simulink model "Quadcopter_State_model_Arduino"  (R2023b)
settings: Solver=VariableStepAuto  StartTime=0.0  StopTime=inf  FixedStep=0.00001  MinStep=0.001  RelTol=1e-3
model workspace (MAT data in the model file):
  DesiredPitchRoll : sugfis (value not decoded)
  DesiredThrust : sugfis (value not decoded)
  DesiredYaw : sugfis (value not decoded)
  Desired_Pitch = 0
  Desired_Roll = 0
  Desired_Yaw = 0
  Desired_Z_Velocity = -3
  FuzzyMotorspeed : sugfis (value not decoded)
values from neighbouring files (symbols this model uses):
  g = 9.81    [Quadcopter_Constants.m]
  Ixx = 0.0294838    [Quadcopter_Constants.m]
  Iyy = 0.0294838    [Quadcopter_Constants.m]
  Izz = 0.058967624    [Quadcopter_Constants.m]
  Jr = (6e-5)*1.358    (= 8.148e-05)    [Quadcopter_Constants.m]
  kd = 1    [Quadcopter_Constants.m]
  kd_phi = 1    [Quadcopter_Constants.m]
  kd_theta = 1    [Quadcopter_Constants.m]
  kf = 1    [Quadcopter_Constants.m]
  ki = 1    [Quadcopter_Constants.m]
  ki_phi = 1    [Quadcopter_Constants.m]
  ki_theta = 1    [Quadcopter_Constants.m]
  km = 4.74157e-9    (= 4.74157e-09)    [Quadcopter_Constants.m]
  kp = 1    [Quadcopter_Constants.m]
  kp_phi = 1    [Quadcopter_Constants.m]
  kp_theta = 1    [Quadcopter_Constants.m]
  kr = (0.1)*1.358    (= 0.1358)    [Quadcopter_Constants.m]
  kt = (0.1)*1.358    (= 0.1358)    [Quadcopter_Constants.m]
  l = 0.254    [Quadcopter_Constants.m]
  m = 0.914    [Quadcopter_Constants.m]
  sample_freq = 1000    [Quadcopter_Constants.m]
undefined symbols (not defined in the file or in its folder): LF
libraries: fuzblock x18, instrumentseriallib x12, simulink_extras x6, vrlib x4, instrumentlib x3, etargetslib x1, slpidlib x1, simulink x1
(part 4 of 5)

== system Quadcopter_State_model_Arduino/Board Fuzzy Only/Fuzzy Control System/Heading Controller ==
  <psi> : Inport
  <psi_dot> : Inport  Port=2
  Bus Creator2 : BusCreator  Inputs=2
  Desired Yaw2 : Constant  Value=Desired_Yaw
  DesiredYaw : fuzblock/Fuzzy Logic  Controller  FIS=DesiredYaw  OutputSampleNumber=101  DataType=double  FuzzifiedInputs=off  RuleFiringStrengths=off  RuleOutputs=off  AggregatedOutputs=off  SimulateUsing=Interpreted execution  OutOfRangeInputValueMessage=warning  NoRuleFiredMessage=warning  EmptyOutputFuzzySetMessage=warning
  Sum3 : Sum  Inputs=|-+
  e_yaw_sat : Saturate  UpperLimit=0.3  LowerLimit=-0.3  OutMin=[-0.3]  OutMax=[0.3]
  psidot_sat : Saturate  UpperLimit=0.3  LowerLimit=-0.3  OutMin=[-0.3]  OutMax=[0.3]
  Desired Yaw1 : Outport
  wires:
  psidot_sat/1 -> Bus Creator2/2
  <psi_dot>/1 -> psidot_sat/1
  Desired Yaw2/1 -> Sum3/2
  e_yaw_sat/1 -> Bus Creator2/1
  <psi>/1 -> Sum3/1
  DesiredYaw/1 -> Desired Yaw1/1  "Desired Yaw"
  Sum3/1 -> e_yaw_sat/1  "e_yaw"
  Bus Creator2/1 -> DesiredYaw/1

== system Quadcopter_State_model_Arduino/Board Fuzzy Only/Fuzzy Control System/Thrust Controller ==
  <z_dot> : Inport
  Desired Thrust : fuzblock/Fuzzy Logic  Controller  FIS=DesiredThrust  OutputSampleNumber=101  DataType=double  FuzzifiedInputs=off  RuleFiringStrengths=off  RuleOutputs=off  AggregatedOutputs=off  SimulateUsing=Interpreted execution  OutOfRangeInputValueMessage=warning  NoRuleFiredMessage=warning  EmptyOutputFuzzySetMessage=warning
  Desired Z Velocity1 : Constant  Value=Desired_Z_Velocity
  Sum : Sum  Inputs=|-+
  e_zdot_sat : Saturate  UpperLimit=0.3  LowerLimit=-0.3  OutMin=[-0.3]  OutMax=[0.3]
  Desired Thrust1 : Outport
  wires:
  Sum/1 -> e_zdot_sat/1  "e_zdot"
  <z_dot>/1 -> Sum/1
  Desired Z Velocity1/1 -> Sum/2
  e_zdot_sat/1 -> Desired Thrust/1
  Desired Thrust/1 -> Desired Thrust1/1  "Desired Thrust"

== system Quadcopter_State_model_Arduino/Board Fuzzy Only/Fuzzy Control System1/Attitude Controller ==
  <phi> : Inport
  <phi_dot> : Inport  Port=2
  <theta> : Inport  Port=3
  <theta_dot> : Inport  Port=4
  Bus Creator1 : BusCreator  Inputs=4
  Demux1 : Demux  Outputs=2
  Desired Pitch2 : Constant  Value=Desired_Pitch
  Desired Roll2 : Constant  Value=Desired_Roll
  DesiredPitchRoll : fuzblock/Fuzzy Logic  Controller  FIS=DesiredPitchRoll  OutputSampleNumber=101  DataType=double  FuzzifiedInputs=off  RuleFiringStrengths=off  RuleOutputs=off  AggregatedOutputs=off  SimulateUsing=Interpreted execution  OutOfRangeInputValueMessage=warning  NoRuleFiredMessage=warning  EmptyOutputFuzzySetMessage=warning
  Sum1 : Sum  Inputs=|-+
  Sum2 : Sum  Inputs=|-+
  e_pitch_sat : Saturate  UpperLimit=0.3  LowerLimit=-0.3  OutMin=[-0.3]  OutMax=[0.3]
  e_roll_sat : Saturate  UpperLimit=0.3  LowerLimit=-0.3  OutMin=[-0.3]  OutMax=[0.3]
  phidot_sat1 : Saturate  UpperLimit=0.3  LowerLimit=-0.3  OutMin=[-0.3]  OutMax=[0.3]
  thetadot_sat : Saturate  UpperLimit=0.3  LowerLimit=-0.3  OutMin=[-0.3]  OutMax=[0.3]
  Desired Roll1 : Outport
  Desired Pitch1 : Outport  Port=2
  wires:
  e_roll_sat/1 -> Bus Creator1/1
  phidot_sat1/1 -> Bus Creator1/4
  Sum2/1 -> e_pitch_sat/1  "e_pitch"
  Desired Roll2/1 -> Sum1/2
  e_pitch_sat/1 -> Bus Creator1/2
  DesiredPitchRoll/1 -> Demux1/1
  Bus Creator1/1 -> DesiredPitchRoll/1
  Demux1/2 -> Desired Pitch1/1  "Desired Pitch"
  Desired Pitch2/1 -> Sum2/2
  Sum1/1 -> e_roll_sat/1  "e_roll"
  thetadot_sat/1 -> Bus Creator1/3
  <phi>/1 -> Sum2/1
  <theta>/1 -> Sum1/1
  Demux1/1 -> Desired Roll1/1  "Desired Roll"
  <phi_dot>/1 -> phidot_sat1/1
  <theta_dot>/1 -> thetadot_sat/1

== system Quadcopter_State_model_Arduino/Board Fuzzy Only/Fuzzy Control System1/Heading Controller ==
  <psi> : Inport
  <psi_dot> : Inport  Port=2
  Bus Creator2 : BusCreator  Inputs=2
  Desired Yaw2 : Constant  Value=Desired_Yaw
  DesiredYaw : fuzblock/Fuzzy Logic  Controller  FIS=DesiredYaw  OutputSampleNumber=101  DataType=double  FuzzifiedInputs=off  RuleFiringStrengths=off  RuleOutputs=off  AggregatedOutputs=off  SimulateUsing=Interpreted execution  OutOfRangeInputValueMessage=warning  NoRuleFiredMessage=warning  EmptyOutputFuzzySetMessage=warning
  Sum3 : Sum  Inputs=|-+
  e_yaw_sat : Saturate  UpperLimit=0.3  LowerLimit=-0.3  OutMin=[-0.3]  OutMax=[0.3]
  psidot_sat : Saturate  UpperLimit=0.3  LowerLimit=-0.3  OutMin=[-0.3]  OutMax=[0.3]
  Desired Yaw1 : Outport
  wires:
  psidot_sat/1 -> Bus Creator2/2
  <psi_dot>/1 -> psidot_sat/1
  Desired Yaw2/1 -> Sum3/2
  e_yaw_sat/1 -> Bus Creator2/1
  <psi>/1 -> Sum3/1
  DesiredYaw/1 -> Desired Yaw1/1  "Desired Yaw"
  Sum3/1 -> e_yaw_sat/1  "e_yaw"
  Bus Creator2/1 -> DesiredYaw/1

== system Quadcopter_State_model_Arduino/Board Fuzzy Only/Fuzzy Control System1/MMA ==
  Desired Thrust1 : Inport
  Desired Yaw1 : Inport  Port=2
  Desired Pitch1 : Inport  Port=3
  Desired Roll1 : Inport  Port=4
  Bus Creator : BusCreator  Inputs=4
  motorspeeds : Outport
  wires:
  Bus Creator/1 -> motorspeeds/1

== system Quadcopter_State_model_Arduino/Board Fuzzy Only/Fuzzy Control System1/Thrust Controller ==
  <z_dot> : Inport
  Desired Thrust : fuzblock/Fuzzy Logic  Controller  FIS=DesiredThrust  OutputSampleNumber=101  DataType=double  FuzzifiedInputs=off  RuleFiringStrengths=off  RuleOutputs=off  AggregatedOutputs=off  SimulateUsing=Interpreted execution  OutOfRangeInputValueMessage=warning  NoRuleFiredMessage=warning  EmptyOutputFuzzySetMessage=warning
  Desired Z Velocity1 : Constant  Value=Desired_Z_Velocity
  Sum : Sum  Inputs=|-+
  e_zdot_sat : Saturate  UpperLimit=2.99999  LowerLimit=-2.99999
  Desired Thrust1 : Outport
  wires:
  Sum/1 -> e_zdot_sat/1  "e_zdot"
  <z_dot>/1 -> Sum/1
  Desired Z Velocity1/1 -> Sum/2
  e_zdot_sat/1 -> Desired Thrust/1
  Desired Thrust/1 -> Desired Thrust1/1  "Desired Thrust"

== system Quadcopter_State_model_Arduino/Board Fuzzy Only/Fuzzy Control System2/Attitude Error ==
  <phi> : Inport
  <phi_dot> : Inport  Port=2
  <theta> : Inport  Port=3
  <theta_dot> : Inport  Port=4
  Desired Pitch2 : Constant  Value=0
  Desired Roll2 : Constant  Value=0
  Sum1 : Sum  Inputs=|-+
  Sum2 : Sum  Inputs=|-+
  e_pitch_sat : Saturate  UpperLimit=0.3  LowerLimit=-0.3  OutMin=[-0.3]  OutMax=[0.3]
  e_roll_sat : Saturate  UpperLimit=0.3  LowerLimit=-0.3  OutMin=[-0.3]  OutMax=[0.3]
  phidot_sat1 : Saturate  UpperLimit=0.3  LowerLimit=-0.3  OutMin=[-0.3]  OutMax=[0.3]
  thetadot_sat : Saturate  UpperLimit=0.3  LowerLimit=-0.3  OutMin=[-0.3]  OutMax=[0.3]
  Out1 : Outport
  Out2 : Outport  Port=2
  Out3 : Outport  Port=3
  Out4 : Outport  Port=4
  wires:
  <phi>/1 -> Sum2/1
  Sum2/1 -> e_pitch_sat/1  "e_pitch"
  Desired Pitch2/1 -> Sum2/2
  <phi_dot>/1 -> phidot_sat1/1
  Desired Roll2/1 -> Sum1/2
  Sum1/1 -> e_roll_sat/1  "e_roll"
  e_pitch_sat/1 -> Out2/1
  <theta_dot>/1 -> thetadot_sat/1
  e_roll_sat/1 -> Out1/1
  <theta>/1 -> Sum1/1
  thetadot_sat/1 -> Out3/1
  phidot_sat1/1 -> Out4/1

== system Quadcopter_State_model_Arduino/Board Fuzzy Only/Fuzzy Control System2/Heading Error ==
  In1 : Inport
  In2 : Inport  Port=2
  Desired Yaw2 : Constant  Value=0
  Sum3 : Sum  Inputs=|-+
  e_yaw_sat : Saturate  UpperLimit=0.3  LowerLimit=-0.3  OutMin=[-0.3]  OutMax=[0.3]
  psidot_sat : Saturate  UpperLimit=0.3  LowerLimit=-0.3  OutMin=[-0.3]  OutMax=[0.3]
  Out1 : Outport
  Out2 : Outport  Port=2
  wires:
  Desired Yaw2/1 -> Sum3/2
  Sum3/1 -> e_yaw_sat/1  "e_yaw"
  In1/1 -> Sum3/1
  e_yaw_sat/1 -> Out1/1
  psidot_sat/1 -> Out2/1
  In2/1 -> psidot_sat/1

== system Quadcopter_State_model_Arduino/Board Fuzzy Only/Fuzzy Control System2/Subsystem ==
  In1 : Inport
  In2 : Inport  Port=2
  Bus Creator1 : BusCreator  Inputs=4
  Demux1 : Demux
  Divide{,1..3} (4 alike) : Product  Inputs=*/
  Gain4 : Gain  Gain=4
  Product{,1..3} (4 alike) : Product
  Scope : Scope  NumInputPorts=4
  Scope1 : Scope  NumInputPorts=4
  Sum : Sum  Inputs=++++  OutDataTypeStr=double  AccumDataTypeStr=double
  Out1 : Outport
  wires:
  In2/1 -> Gain4/1
  Demux1/2 -> Sum/2, Scope/2, Divide3/1  "Omega2"
  Divide1/1 -> Product3/1
  Sum/1 -> Divide1/2, Divide2/2, Divide3/2, Divide/2
  Demux1/1 -> Sum/1, Divide/1, Scope/1  "Omega1"
  Demux1/4 -> Sum/4, Scope/4, Divide1/1  "Omega4"
  Divide3/1 -> Product1/1
  Divide/1 -> Product/1
  Bus Creator1/1 -> Out1/1
  Demux1/3 -> Scope/3, Divide2/1, Sum/3  "Omega3"
  Divide2/1 -> Product2/1
  In1/1 -> Demux1/1
  Product/1 -> Scope1/1, Bus Creator1/1
  Product1/1 -> Scope1/2, Bus Creator1/2
  Product2/1 -> Scope1/3, Bus Creator1/3
  Product3/1 -> Scope1/4, Bus Creator1/4
  Gain4/1 -> Product3/2, Product2/2, Product1/2, Product/2

== system Quadcopter_State_model_Arduino/Board Fuzzy Only/Fuzzy Control System2/Zdot Error ==
  In1 : Inport
  Desired Z Velocity1 : Constant  Value=0
  Sum : Sum  Inputs=|-+
  e_zdot_sat : Saturate  UpperLimit=3  LowerLimit=-3  OutMin=[-3]  OutMax=[3]
  Out1 : Outport
  wires:
  In1/1 -> Sum/1
  Sum/1 -> e_zdot_sat/1  "e_zdot"
  Desired Z Velocity1/1 -> Sum/2
  e_zdot_sat/1 -> Out1/1

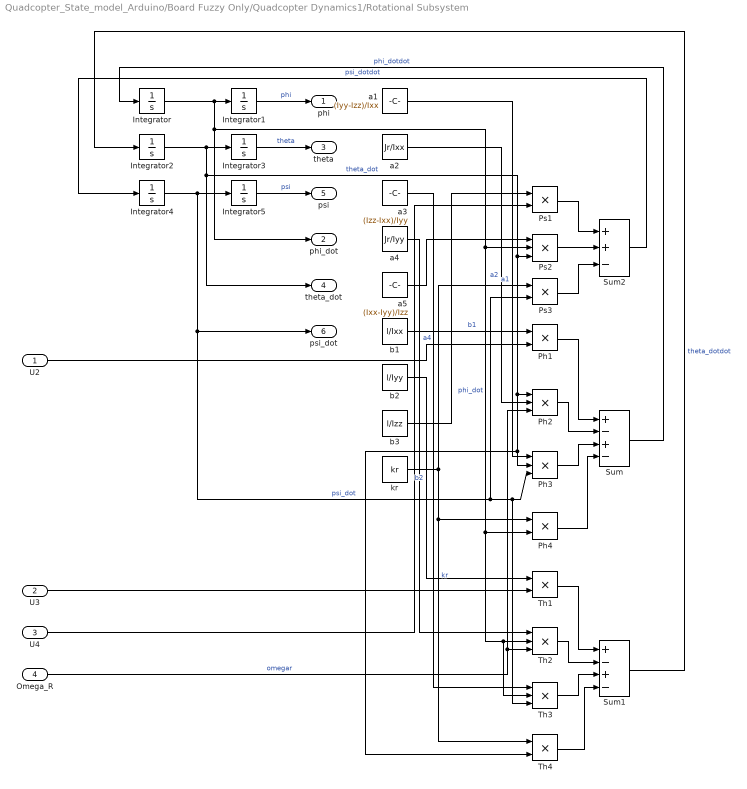
== system Quadcopter_State_model_Arduino/Board Fuzzy Only/Quadcopter Dynamics1/Rotational Subsystem ==
  U2 : Inport
  U3 : Inport  Port=2
  U4 : Inport  Port=3
  Omega_R : Inport  Port=4
  Integrator{,1..5} (6 alike) : Integrator
  Ph1 : Product
  Ph2 : Product  Inputs=3
  Ph3 : Product  Inputs=3
  Ph4 : Product
  Ps1 : Product
  Ps2 : Product  Inputs=3
  Ps3 : Product
  Sum : Sum  Inputs=+-+-
  Sum1 : Sum  Inputs=+-+-
  Sum2 : Sum  Inputs=++-
  Th1 : Product
  Th2 : Product  Inputs=3
  Th3 : Product  Inputs=3
  Th4 : Product
  a1 : Constant  Value=(Iyy-Izz)/Ixx
  a2 : Constant  Value=Jr/Ixx
  a3 : Constant  Value=(Izz-Ixx)/Iyy
  a4 : Constant  Value=Jr/Iyy
  a5 : Constant  Value=(Ixx-Iyy)/Izz
  b1 : Constant  Value=l/Ixx
  b2 : Constant  Value=l/Iyy
  b3 : Constant  Value=l/Izz
  kr : Constant  Value=kr
  phi : Outport
  phi_dot : Outport  Port=2
  theta : Outport  Port=3
  theta_dot : Outport  Port=4
  psi : Outport  Port=5
  psi_dot : Outport  Port=6
  wires:
  U4/1 -> Ps1/2
  Ph3/1 -> Sum/3
  kr/1 -> Ps3/1, Ph4/1, Th4/1  "kr"
  Th1/1 -> Sum1/1
  Sum/1 -> Integrator/1  "phi_dotdot"
  Omega_R/1 -> Ph2/3, Th2/3  "omegar"
  Th2/1 -> Sum1/2
  Integrator4/1 -> Integrator5/1, psi_dot/1, Ps3/2, Th3/3, Ph3/3  "psi_dot"
  Integrator2/1 -> Integrator3/1, theta_dot/1, Ps2/3, Ph3/2, Th4/2, Ph2/1  "theta_dot"
  Th3/1 -> Sum1/3
  a4/1 -> Th2/1  "a4"
  Sum2/1 -> Integrator4/1  "psi_dotdot"
  Integrator1/1 -> phi/1  "phi"
  U2/1 -> Ph1/2
  Sum1/1 -> Integrator2/1  "theta_dotdot"
  Integrator/1 -> phi_dot/1, Ps2/2, Ph4/2, Th3/2, Th2/2, Integrator1/1  "phi_dot"
  Th4/1 -> Sum1/4
  Integrator3/1 -> theta/1  "theta"
  b1/1 -> Ph1/1  "b1"
  a3/1 -> Th3/1
  b3/1 -> Ps1/1
  a2/1 -> Ph2/2  "a2"
  a1/1 -> Ph3/1  "a1"
  a5/1 -> Ps2/1
  U3/1 -> Th1/2
  Ps3/1 -> Sum2/3
  Ps1/1 -> Sum2/1
  Ps2/1 -> Sum2/2
  Ph4/1 -> Sum/4
  b2/1 -> Th1/1  "b2"
  Ph1/1 -> Sum/1
  Ph2/1 -> Sum/2
  Integrator5/1 -> psi/1  "psi"

== system Quadcopter_State_model_Arduino/Board Fuzzy Only/Quadcopter Dynamics1/Translational Subsystem 2.0 ==
  U1 : Inport
  phi : Inport  Port=2
  theta : Inport  Port=3
  psi : Inport  Port=4
  FWx : Inport  Port=5
  FWy : Inport  Port=6
  FWz : Inport  Port=7
  Integrator{6..11} (6 alike) : Integrator
  x_dotdot : Subsystem
      settings: PortSchema="{\"entries\":[{\"content\":{\"sides\":[{\"content\":{\"connectorIds\":[\"In1\",\"In2\",\"In3\",\"In4\",\"In5\",\"In6\",\"In7\"]},\"type\":\"ConnectorPlacement.EquallySpacedRectSide\",\"uuid\":\"e18be740-6f58-4938-bfd9-cb9ac7dcd4da\"},{\"content\":{\"connectorIds\":[\"In8\",\"Out1\"],\"side\":\"RIGHT\"},\"type\":\"ConnectorPlacement.EquallySpacedRectSide\",\"uuid\":\"68bb1cbd-6e96-465a-bd08-5b84ec49c8af\"},{\"content\":{\"connectorIds\":[],\"side\":\"TOP\"},\"type\":\"ConnectorPlacement.EquallySpacedRectSide\",\"uuid\":\"38ea75c0-d618-4b9d-8119-0da292fc369a\"}]},\"type\":\"ConnectorPlacement.EquallySpacedConnector\",\"uuid\":\"3f5248e6-8959-4c7a-b37c-028caf22ec16\"}],\"packageUris\":[\"http://schema.mathworks.com/mf0/Connector/R2020b\"],\"version\":\"1.0\"}"
  y_dotdot : Subsystem
      settings: PortSchema="{\"entries\":[{\"content\":{\"sides\":[{\"content\":{\"connectorIds\":[\"In1\",\"In2\",\"In3\",\"In4\",\"In5\",\"In6\",\"In7\"]},\"type\":\"ConnectorPlacement.EquallySpacedRectSide\",\"uuid\":\"e18be740-6f58-4938-bfd9-cb9ac7dcd4da\"},{\"content\":{\"connectorIds\":[\"In8\",\"Out1\"],\"side\":\"RIGHT\"},\"type\":\"ConnectorPlacement.EquallySpacedRectSide\",\"uuid\":\"68bb1cbd-6e96-465a-bd08-5b84ec49c8af\"},{\"content\":{\"connectorIds\":[],\"side\":\"TOP\"},\"type\":\"ConnectorPlacement.EquallySpacedRectSide\",\"uuid\":\"38ea75c0-d618-4b9d-8119-0da292fc369a\"}]},\"type\":\"ConnectorPlacement.EquallySpacedConnector\",\"uuid\":\"3f5248e6-8959-4c7a-b37c-028caf22ec16\"}],\"packageUris\":[\"http://schema.mathworks.com/mf0/Connector/R2020b\"],\"version\":\"1.0\"}"
  z_dodot : Subsystem
      settings: PortSchema="{\"entries\":[{\"content\":{\"sides\":[{\"content\":{\"connectorIds\":[\"In1\",\"In2\",\"In3\",\"In4\",\"In5\",\"In6\"]},\"type\":\"ConnectorPlacement.EquallySpacedRectSide\",\"uuid\":\"469c81c2-5293-4bed-8306-2e0ffdc3049a\"},{\"content\":{\"connectorIds\":[\"In7\",\"Out1\"],\"side\":\"RIGHT\"},\"type\":\"ConnectorPlacement.EquallySpacedRectSide\",\"uuid\":\"eb4ccd77-d780-4218-b458-09af15aced4a\"},{\"content\":{\"connectorIds\":[],\"side\":\"TOP\"},\"type\":\"ConnectorPlacement.EquallySpacedRectSide\",\"uuid\":\"6490e6c2-4333-4700-a2fe-e5c918a55a4d\"}]},\"type\":\"ConnectorPlacement.EquallySpacedConnector\",\"uuid\":\"88d53b3a-6da6-4ffe-908b-5dd465569eed\"}],\"packageUris\":[\"http://schema.mathworks.com/mf0/Connector/R2020b\"],\"version\":\"1.0\"}"
  x : Outport
  x_dot : Outport  Port=2
  y : Outport  Port=3
  y_dot : Outport  Port=4
  z : Outport  Port=5
  z_dot : Outport  Port=6
  wires:
  Integrator10/1 -> z_dot/1, z_dodot/7(z_dot), Integrator11/1  "z_dot"
  Integrator8/1 -> Integrator9/1, y_dotdot/8(y_dot), y_dot/1  "y_dot"
  Integrator9/1 -> y/1  "y"
  Integrator7/1 -> x/1  "x"
  Integrator6/1 -> x_dotdot/8(x_dot), x_dot/1, Integrator7/1  "x_dot"
  Integrator11/1 -> z/1  "z"
  U1/1 -> z_dodot/1(U1), y_dotdot/1(U1), x_dotdot/1(U1)  "U1"
  phi/1 -> y_dotdot/2(phi), x_dotdot/2(phi), z_dodot/2(phi)  "Phi"
  theta/1 -> z_dodot/3(theta), y_dotdot/3(theta), x_dotdot/3(theta)  "Theta"
  psi/1 -> y_dotdot/4(psi), x_dotdot/4(psi)  "Psi"
  FWx/1 -> z_dodot/4(FWx), y_dotdot/5(FWx), x_dotdot/5(FWx)  "FWx"
  FWy/1 -> z_dodot/5(FWy), y_dotdot/6(FWy), x_dotdot/6(FWy)  "FWy"
  FWz/1 -> z_dodot/6(FWz), y_dotdot/7(FWz), x_dotdot/7(FWz)  "FWz"
  z_dodot/1(z_dotdot) -> Integrator10/1
  y_dotdot/1(y_dotdot) -> Integrator8/1
  x_dotdot/1(x_dotdot) -> Integrator6/1

== system Quadcopter_State_model_Arduino/Board Fuzzy Only/Quadcopter Dynamics1/Translational Wind Engine ==
  phi : Inport
  theta : Inport  Port=2
  psi : Inport  Port=3
  Projected Areas : Subsystem
  Wind Forces : Subsystem
  Wind Generation : Subsystem
  FWx : Outport
  FWy : Outport  Port=2
  FWz : Outport  Port=3
  wires:
  theta/1 -> Projected Areas/1(theta)
  Wind Generation/3(VWz) -> Wind Forces/6(VWz)
  Projected Areas/3(Az) -> Wind Forces/3(Az)
  Wind Forces/3(FWz) -> FWz/1
  Wind Generation/2(VWy) -> Wind Forces/5(VWy)
  Projected Areas/1(Ax) -> Wind Forces/1(Ax)
  Projected Areas/2(Ay) -> Wind Forces/2(Ay)
  Wind Generation/1(VWx) -> Wind Forces/4(VWx)
  phi/1 -> Projected Areas/3(phi)
  psi/1 -> Projected Areas/2(psi)
  Wind Forces/2(FWy) -> FWy/1
  Wind Forces/1(FWx) -> FWx/1

== system Quadcopter_State_model_Arduino/Fuzzy Simulation/Fuzzy Control System/Attitude Controller ==
  <phi> : Inport
  <phi_dot> : Inport  Port=2
  <theta> : Inport  Port=3
  <theta_dot> : Inport  Port=4
  Bus Creator1 : BusCreator  Inputs=4
  Demux1 : Demux  Outputs=2
  Desired Pitch2 : Constant  Value=Desired_Pitch
  Desired Roll2 : Constant  Value=Desired_Roll
  DesiredPitchRoll : fuzblock/Fuzzy Logic  Controller  FIS=DesiredPitchRoll  OutputSampleNumber=101  DataType=double  FuzzifiedInputs=off  RuleFiringStrengths=off  RuleOutputs=off  AggregatedOutputs=off  SimulateUsing=Interpreted execution  OutOfRangeInputValueMessage=warning  NoRuleFiredMessage=warning  EmptyOutputFuzzySetMessage=warning
  Sum1 : Sum  Inputs=|-+
  Sum2 : Sum  Inputs=|-+
  e_pitch_sat : Saturate  UpperLimit=0.3  LowerLimit=-0.3  OutMin=[-0.3]  OutMax=[0.3]
  e_roll_sat : Saturate  UpperLimit=0.3  LowerLimit=-0.3  OutMin=[-0.3]  OutMax=[0.3]
  phidot_sat1 : Saturate  UpperLimit=0.3  LowerLimit=-0.3  OutMin=[-0.3]  OutMax=[0.3]
  thetadot_sat : Saturate  UpperLimit=0.3  LowerLimit=-0.3  OutMin=[-0.3]  OutMax=[0.3]
  Desired Roll1 : Outport
  Desired Pitch1 : Outport  Port=2
  wires:
  e_roll_sat/1 -> Bus Creator1/1
  phidot_sat1/1 -> Bus Creator1/4
  Sum2/1 -> e_pitch_sat/1  "e_pitch"
  Desired Roll2/1 -> Sum1/2
  e_pitch_sat/1 -> Bus Creator1/2
  DesiredPitchRoll/1 -> Demux1/1
  Bus Creator1/1 -> DesiredPitchRoll/1
  Demux1/2 -> Desired Pitch1/1  "Desired Pitch"
  Desired Pitch2/1 -> Sum2/2
  Sum1/1 -> e_roll_sat/1  "e_roll"
  thetadot_sat/1 -> Bus Creator1/3
  <phi>/1 -> Sum2/1
  <theta>/1 -> Sum1/1
  Demux1/1 -> Desired Roll1/1  "Desired Roll"
  <phi_dot>/1 -> phidot_sat1/1
  <theta_dot>/1 -> thetadot_sat/1

== system Quadcopter_State_model_Arduino/Fuzzy Simulation/Fuzzy Control System/Heading Controller ==
  <psi> : Inport
  <psi_dot> : Inport  Port=2
  Bus Creator2 : BusCreator  Inputs=2
  Desired Yaw2 : Constant  Value=Desired_Yaw
  DesiredYaw : fuzblock/Fuzzy Logic  Controller  FIS=DesiredYaw  OutputSampleNumber=101  DataType=double  FuzzifiedInputs=off  RuleFiringStrengths=off  RuleOutputs=off  AggregatedOutputs=off  SimulateUsing=Interpreted execution  OutOfRangeInputValueMessage=warning  NoRuleFiredMessage=warning  EmptyOutputFuzzySetMessage=warning
  Sum3 : Sum  Inputs=|-+
  e_yaw_sat : Saturate  UpperLimit=0.3  LowerLimit=-0.3  OutMin=[-0.3]  OutMax=[0.3]
  psidot_sat : Saturate  UpperLimit=0.3  LowerLimit=-0.3  OutMin=[-0.3]  OutMax=[0.3]
  Desired Yaw1 : Outport
  wires:
  psidot_sat/1 -> Bus Creator2/2
  <psi_dot>/1 -> psidot_sat/1
  Desired Yaw2/1 -> Sum3/2
  e_yaw_sat/1 -> Bus Creator2/1
  <psi>/1 -> Sum3/1
  DesiredYaw/1 -> Desired Yaw1/1  "Desired Yaw"
  Sum3/1 -> e_yaw_sat/1  "e_yaw"
  Bus Creator2/1 -> DesiredYaw/1

== system Quadcopter_State_model_Arduino/Fuzzy Simulation/Fuzzy Control System/Thrust Controller ==
  <z_dot> : Inport
  Desired Thrust : fuzblock/Fuzzy Logic  Controller  FIS=DesiredThrust  OutputSampleNumber=101  DataType=double  FuzzifiedInputs=off  RuleFiringStrengths=off  RuleOutputs=off  AggregatedOutputs=off  SimulateUsing=Interpreted execution  OutOfRangeInputValueMessage=warning  NoRuleFiredMessage=warning  EmptyOutputFuzzySetMessage=warning
  Desired Z Velocity1 : Constant  Value=Desired_Z_Velocity
  Sum : Sum  Inputs=|-+
  e_zdot_sat : Saturate  UpperLimit=0.3  LowerLimit=-0.3  OutMin=[-0.3]  OutMax=[0.3]
  Desired Thrust1 : Outport
  wires:
  Sum/1 -> e_zdot_sat/1  "e_zdot"
  <z_dot>/1 -> Sum/1
  Desired Z Velocity1/1 -> Sum/2
  e_zdot_sat/1 -> Desired Thrust/1
  Desired Thrust/1 -> Desired Thrust1/1  "Desired Thrust"

== system Quadcopter_State_model_Arduino/Fuzzy Simulation/Fuzzy Control System1/Attitude Controller ==
  <phi> : Inport
  <phi_dot> : Inport  Port=2
  <theta> : Inport  Port=3
  <theta_dot> : Inport  Port=4
  Bus Creator1 : BusCreator  Inputs=4
  Demux1 : Demux  Outputs=2
  Desired Pitch2 : Constant  Value=Desired_Pitch
  Desired Roll2 : Constant  Value=Desired_Roll
  DesiredPitchRoll : fuzblock/Fuzzy Logic  Controller  FIS=DesiredPitchRoll  OutputSampleNumber=101  DataType=double  FuzzifiedInputs=off  RuleFiringStrengths=off  RuleOutputs=off  AggregatedOutputs=off  SimulateUsing=Interpreted execution  OutOfRangeInputValueMessage=warning  NoRuleFiredMessage=warning  EmptyOutputFuzzySetMessage=warning
  Sum1 : Sum  Inputs=|-+
  Sum2 : Sum  Inputs=|-+
  e_pitch_sat : Saturate  UpperLimit=0.3  LowerLimit=-0.3  OutMin=[-0.3]  OutMax=[0.3]
  e_roll_sat : Saturate  UpperLimit=0.3  LowerLimit=-0.3  OutMin=[-0.3]  OutMax=[0.3]
  phidot_sat1 : Saturate  UpperLimit=0.3  LowerLimit=-0.3  OutMin=[-0.3]  OutMax=[0.3]
  thetadot_sat : Saturate  UpperLimit=0.3  LowerLimit=-0.3  OutMin=[-0.3]  OutMax=[0.3]
  Desired Roll1 : Outport
  Desired Pitch1 : Outport  Port=2
  wires:
  e_roll_sat/1 -> Bus Creator1/1
  phidot_sat1/1 -> Bus Creator1/4
  Sum2/1 -> e_pitch_sat/1  "e_pitch"
  Desired Roll2/1 -> Sum1/2
  e_pitch_sat/1 -> Bus Creator1/2
  DesiredPitchRoll/1 -> Demux1/1
  Bus Creator1/1 -> DesiredPitchRoll/1
  Demux1/2 -> Desired Pitch1/1  "Desired Pitch"
  Desired Pitch2/1 -> Sum2/2
  Sum1/1 -> e_roll_sat/1  "e_roll"
  thetadot_sat/1 -> Bus Creator1/3
  <phi>/1 -> Sum2/1
  <theta>/1 -> Sum1/1
  Demux1/1 -> Desired Roll1/1  "Desired Roll"
  <phi_dot>/1 -> phidot_sat1/1
  <theta_dot>/1 -> thetadot_sat/1

== system Quadcopter_State_model_Arduino/Fuzzy Simulation/Fuzzy Control System1/Heading Controller ==
  <psi> : Inport
  <psi_dot> : Inport  Port=2
  Bus Creator2 : BusCreator  Inputs=2
  Desired Yaw2 : Constant  Value=Desired_Yaw
  DesiredYaw : fuzblock/Fuzzy Logic  Controller  FIS=DesiredYaw  OutputSampleNumber=101  DataType=double  FuzzifiedInputs=off  RuleFiringStrengths=off  RuleOutputs=off  AggregatedOutputs=off  SimulateUsing=Interpreted execution  OutOfRangeInputValueMessage=warning  NoRuleFiredMessage=warning  EmptyOutputFuzzySetMessage=warning
  Sum3 : Sum  Inputs=|-+
  e_yaw_sat : Saturate  UpperLimit=0.3  LowerLimit=-0.3  OutMin=[-0.3]  OutMax=[0.3]
  psidot_sat : Saturate  UpperLimit=0.3  LowerLimit=-0.3  OutMin=[-0.3]  OutMax=[0.3]
  Desired Yaw1 : Outport
  wires:
  psidot_sat/1 -> Bus Creator2/2
  <psi_dot>/1 -> psidot_sat/1
  Desired Yaw2/1 -> Sum3/2
  e_yaw_sat/1 -> Bus Creator2/1
  <psi>/1 -> Sum3/1
  DesiredYaw/1 -> Desired Yaw1/1  "Desired Yaw"
  Sum3/1 -> e_yaw_sat/1  "e_yaw"
  Bus Creator2/1 -> DesiredYaw/1

== system Quadcopter_State_model_Arduino/Fuzzy Simulation/Fuzzy Control System1/MMA ==
  Desired Thrust1 : Inport
  Desired Yaw1 : Inport  Port=2
  Desired Pitch1 : Inport  Port=3
  Desired Roll1 : Inport  Port=4
  Bus Creator : BusCreator  Inputs=4
  motorspeeds : Outport
  wires:
  Bus Creator/1 -> motorspeeds/1

== system Quadcopter_State_model_Arduino/Fuzzy Simulation/Fuzzy Control System1/Thrust Controller ==
  <z_dot> : Inport
  Desired Thrust : fuzblock/Fuzzy Logic  Controller  FIS=DesiredThrust  OutputSampleNumber=101  DataType=double  FuzzifiedInputs=off  RuleFiringStrengths=off  RuleOutputs=off  AggregatedOutputs=off  SimulateUsing=Interpreted execution  OutOfRangeInputValueMessage=warning  NoRuleFiredMessage=warning  EmptyOutputFuzzySetMessage=warning
  Desired Z Velocity1 : Constant  Value=Desired_Z_Velocity
  Sum : Sum  Inputs=|-+
  e_zdot_sat : Saturate  UpperLimit=2.99999  LowerLimit=-2.99999
  Desired Thrust1 : Outport
  wires:
  Sum/1 -> e_zdot_sat/1  "e_zdot"
  <z_dot>/1 -> Sum/1
  Desired Z Velocity1/1 -> Sum/2
  e_zdot_sat/1 -> Desired Thrust/1
  Desired Thrust/1 -> Desired Thrust1/1  "Desired Thrust"

== system Quadcopter_State_model_Arduino/Fuzzy Simulation/Fuzzy Control System2/Attitude Controller ==
  <phi> : Inport
  <phi_dot> : Inport  Port=2
  <theta> : Inport  Port=3
  <theta_dot> : Inport  Port=4
  Bus Creator1 : BusCreator  Inputs=4
  Demux1 : Demux  Outputs=2
  Desired Pitch2 : Constant  Value=0
  Desired Roll2 : Constant  Value=-0.3
  DesiredPitchRoll : fuzblock/Fuzzy Logic  Controller  FIS=DesiredPitchRoll  OutputSampleNumber=101  DataType=double  FuzzifiedInputs=off  RuleFiringStrengths=off  RuleOutputs=off  AggregatedOutputs=off  SimulateUsing=Interpreted execution  OutOfRangeInputValueMessage=warning  NoRuleFiredMessage=warning  EmptyOutputFuzzySetMessage=warning
  Sum1 : Sum  Inputs=|-+
  Sum2 : Sum  Inputs=|-+
  e_pitch_sat : Saturate  UpperLimit=0.3  LowerLimit=-0.3  OutMin=[-0.3]  OutMax=[0.3]
  e_roll_sat : Saturate  UpperLimit=0.3  LowerLimit=-0.3  OutMin=[-0.3]  OutMax=[0.3]
  phidot_sat1 : Saturate  UpperLimit=0.3  LowerLimit=-0.3  OutMin=[-0.3]  OutMax=[0.3]
  thetadot_sat : Saturate  UpperLimit=0.3  LowerLimit=-0.3  OutMin=[-0.3]  OutMax=[0.3]
  Desired Roll1 : Outport
  Desired Pitch1 : Outport  Port=2
  wires:
  e_roll_sat/1 -> Bus Creator1/1
  phidot_sat1/1 -> Bus Creator1/4
  Sum2/1 -> e_pitch_sat/1  "e_pitch"
  Desired Roll2/1 -> Sum1/2
  e_pitch_sat/1 -> Bus Creator1/2
  DesiredPitchRoll/1 -> Demux1/1
  Bus Creator1/1 -> DesiredPitchRoll/1
  Demux1/2 -> Desired Pitch1/1  "Desired Pitch"
  Desired Pitch2/1 -> Sum2/2
  Sum1/1 -> e_roll_sat/1  "e_roll"
  thetadot_sat/1 -> Bus Creator1/3
  <phi>/1 -> Sum2/1
  <theta>/1 -> Sum1/1
  Demux1/1 -> Desired Roll1/1  "Desired Roll"
  <phi_dot>/1 -> phidot_sat1/1
  <theta_dot>/1 -> thetadot_sat/1

== system Quadcopter_State_model_Arduino/Fuzzy Simulation/Fuzzy Control System2/Heading Controller ==
  <psi> : Inport
  <psi_dot> : Inport  Port=2
  Bus Creator2 : BusCreator  Inputs=2
  Desired Yaw2 : Constant  Value=0
  DesiredYaw : fuzblock/Fuzzy Logic  Controller  FIS=DesiredYaw  OutputSampleNumber=101  DataType=double  FuzzifiedInputs=off  RuleFiringStrengths=off  RuleOutputs=off  AggregatedOutputs=off  SimulateUsing=Interpreted execution  OutOfRangeInputValueMessage=warning  NoRuleFiredMessage=warning  EmptyOutputFuzzySetMessage=warning
  Sum3 : Sum  Inputs=|-+
  e_yaw_sat : Saturate  UpperLimit=0.3  LowerLimit=-0.3  OutMin=[-0.3]  OutMax=[0.3]
  psidot_sat : Saturate  UpperLimit=0.3  LowerLimit=-0.3  OutMin=[-0.3]  OutMax=[0.3]
  Desired Yaw1 : Outport
  wires:
  psidot_sat/1 -> Bus Creator2/2
  <psi_dot>/1 -> psidot_sat/1
  Desired Yaw2/1 -> Sum3/2
  e_yaw_sat/1 -> Bus Creator2/1
  <psi>/1 -> Sum3/1
  DesiredYaw/1 -> Desired Yaw1/1  "Desired Yaw"
  Sum3/1 -> e_yaw_sat/1  "e_yaw"
  Bus Creator2/1 -> DesiredYaw/1

== system Quadcopter_State_model_Arduino/Fuzzy Simulation/Fuzzy Control System2/Subsystem ==
  In1 : Inport
  In2 : Inport  Port=2
  Bus Creator1 : BusCreator  Inputs=4
  Demux1 : Demux
  Divide{,1..3} (4 alike) : Product  Inputs=*/
  Gain4 : Gain  Gain=4
  Product{,1..3} (4 alike) : Product
  Scope : Scope  NumInputPorts=4
  Scope1 : Scope  NumInputPorts=4
  Sum : Sum  Inputs=++++
  Out1 : Outport
  wires:
  In2/1 -> Gain4/1
  Demux1/2 -> Sum/2, Scope/2, Divide3/1  "Omega2"
  Divide1/1 -> Product3/1
  Sum/1 -> Divide1/2, Divide2/2, Divide3/2, Divide/2
  Demux1/1 -> Sum/1, Divide/1, Scope/1  "Omega1"
  Demux1/4 -> Sum/4, Scope/4, Divide1/1  "Omega4"
  Divide3/1 -> Product1/1
  Divide/1 -> Product/1
  Bus Creator1/1 -> Out1/1
  Demux1/3 -> Scope/3, Divide2/1, Sum/3  "Omega3"
  Divide2/1 -> Product2/1
  In1/1 -> Demux1/1
  Product/1 -> Scope1/1, Bus Creator1/1
  Product1/1 -> Scope1/2, Bus Creator1/2
  Product2/1 -> Scope1/3, Bus Creator1/3
  Product3/1 -> Scope1/4, Bus Creator1/4
  Gain4/1 -> Product3/2, Product2/2, Product1/2, Product/2

== system Quadcopter_State_model_Arduino/Fuzzy Simulation/Fuzzy Control System2/Thrust Controller ==
  <z_dot> : Inport
  Desired Thrust : fuzblock/Fuzzy Logic  Controller  FIS=DesiredThrust  OutputSampleNumber=101  DataType=double  FuzzifiedInputs=off  RuleFiringStrengths=off  RuleOutputs=off  AggregatedOutputs=off  SimulateUsing=Interpreted execution  OutOfRangeInputValueMessage=warning  NoRuleFiredMessage=warning  EmptyOutputFuzzySetMessage=warning
  Desired Z Velocity1 : Constant  Value=0
  Gain : Gain  Gain=1.36
  Saturation : Saturate  UpperLimit=255  LowerLimit=0  OutMin=[0]  OutMax=[255]
  Sum : Sum  Inputs=|-+
  e_zdot_sat : Saturate  UpperLimit=0.3  LowerLimit=-0.3  OutMin=[-0.3]  OutMax=[0.3]
  Desired Thrust1 : Outport
  wires:
  Sum/1 -> e_zdot_sat/1  "e_zdot"
  <z_dot>/1 -> Sum/1
  Desired Z Velocity1/1 -> Sum/2
  e_zdot_sat/1 -> Desired Thrust/1
  Desired Thrust/1 -> Gain/1  "Desired Thrust"
  Gain/1 -> Saturation/1
  Saturation/1 -> Desired Thrust1/1

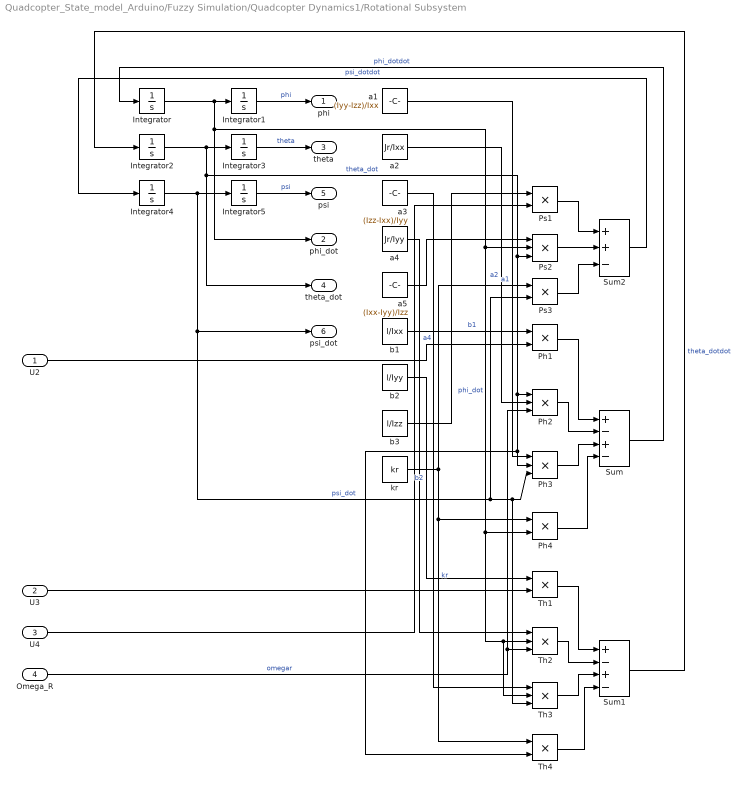
== system Quadcopter_State_model_Arduino/Fuzzy Simulation/Quadcopter Dynamics1/Rotational Subsystem ==
  U2 : Inport
  U3 : Inport  Port=2
  U4 : Inport  Port=3
  Omega_R : Inport  Port=4
  Integrator{,1..5} (6 alike) : Integrator
  Ph1 : Product
  Ph2 : Product  Inputs=3
  Ph3 : Product  Inputs=3
  Ph4 : Product
  Ps1 : Product
  Ps2 : Product  Inputs=3
  Ps3 : Product
  Sum : Sum  Inputs=+-+-
  Sum1 : Sum  Inputs=+-+-
  Sum2 : Sum  Inputs=++-
  Th1 : Product
  Th2 : Product  Inputs=3
  Th3 : Product  Inputs=3
  Th4 : Product
  a1 : Constant  Value=(Iyy-Izz)/Ixx
  a2 : Constant  Value=Jr/Ixx
  a3 : Constant  Value=(Izz-Ixx)/Iyy
  a4 : Constant  Value=Jr/Iyy
  a5 : Constant  Value=(Ixx-Iyy)/Izz
  b1 : Constant  Value=l/Ixx
  b2 : Constant  Value=l/Iyy
  b3 : Constant  Value=l/Izz
  kr : Constant  Value=kr
  phi : Outport
  phi_dot : Outport  Port=2
  theta : Outport  Port=3
  theta_dot : Outport  Port=4
  psi : Outport  Port=5
  psi_dot : Outport  Port=6
  wires:
  U4/1 -> Ps1/2
  Ph3/1 -> Sum/3
  kr/1 -> Ps3/1, Ph4/1, Th4/1  "kr"
  Th1/1 -> Sum1/1
  Sum/1 -> Integrator/1  "phi_dotdot"
  Omega_R/1 -> Ph2/3, Th2/3  "omegar"
  Th2/1 -> Sum1/2
  Integrator4/1 -> Integrator5/1, psi_dot/1, Ps3/2, Th3/3, Ph3/3  "psi_dot"
  Integrator2/1 -> Integrator3/1, theta_dot/1, Ps2/3, Ph3/2, Th4/2, Ph2/1  "theta_dot"
  Th3/1 -> Sum1/3
  a4/1 -> Th2/1  "a4"
  Sum2/1 -> Integrator4/1  "psi_dotdot"
  Integrator1/1 -> phi/1  "phi"
  U2/1 -> Ph1/2
  Sum1/1 -> Integrator2/1  "theta_dotdot"
  Integrator/1 -> phi_dot/1, Ps2/2, Ph4/2, Th3/2, Th2/2, Integrator1/1  "phi_dot"
  Th4/1 -> Sum1/4
  Integrator3/1 -> theta/1  "theta"
  b1/1 -> Ph1/1  "b1"
  a3/1 -> Th3/1
  b3/1 -> Ps1/1
  a2/1 -> Ph2/2  "a2"
  a1/1 -> Ph3/1  "a1"
  a5/1 -> Ps2/1
  U3/1 -> Th1/2
  Ps3/1 -> Sum2/3
  Ps1/1 -> Sum2/1
  Ps2/1 -> Sum2/2
  Ph4/1 -> Sum/4
  b2/1 -> Th1/1  "b2"
  Ph1/1 -> Sum/1
  Ph2/1 -> Sum/2
  Integrator5/1 -> psi/1  "psi"

== system Quadcopter_State_model_Arduino/Fuzzy Simulation/Quadcopter Dynamics1/Translational Subsystem 2.0 ==
  U1 : Inport
  phi : Inport  Port=2
  theta : Inport  Port=3
  psi : Inport  Port=4
  FWx : Inport  Port=5
  FWy : Inport  Port=6
  FWz : Inport  Port=7
  Integrator{6..11} (6 alike) : Integrator
  x_dotdot : Subsystem
      settings: PortSchema="{\"entries\":[{\"content\":{\"sides\":[{\"content\":{\"connectorIds\":[\"In1\",\"In2\",\"In3\",\"In4\",\"In5\",\"In6\",\"In7\"]},\"type\":\"ConnectorPlacement.EquallySpacedRectSide\",\"uuid\":\"e18be740-6f58-4938-bfd9-cb9ac7dcd4da\"},{\"content\":{\"connectorIds\":[\"In8\",\"Out1\"],\"side\":\"RIGHT\"},\"type\":\"ConnectorPlacement.EquallySpacedRectSide\",\"uuid\":\"68bb1cbd-6e96-465a-bd08-5b84ec49c8af\"},{\"content\":{\"connectorIds\":[],\"side\":\"TOP\"},\"type\":\"ConnectorPlacement.EquallySpacedRectSide\",\"uuid\":\"38ea75c0-d618-4b9d-8119-0da292fc369a\"}]},\"type\":\"ConnectorPlacement.EquallySpacedConnector\",\"uuid\":\"3f5248e6-8959-4c7a-b37c-028caf22ec16\"}],\"packageUris\":[\"http://schema.mathworks.com/mf0/Connector/R2020b\"],\"version\":\"1.0\"}"
  y_dotdot : Subsystem
      settings: PortSchema="{\"entries\":[{\"content\":{\"sides\":[{\"content\":{\"connectorIds\":[\"In1\",\"In2\",\"In3\",\"In4\",\"In5\",\"In6\",\"In7\"]},\"type\":\"ConnectorPlacement.EquallySpacedRectSide\",\"uuid\":\"e18be740-6f58-4938-bfd9-cb9ac7dcd4da\"},{\"content\":{\"connectorIds\":[\"In8\",\"Out1\"],\"side\":\"RIGHT\"},\"type\":\"ConnectorPlacement.EquallySpacedRectSide\",\"uuid\":\"68bb1cbd-6e96-465a-bd08-5b84ec49c8af\"},{\"content\":{\"connectorIds\":[],\"side\":\"TOP\"},\"type\":\"ConnectorPlacement.EquallySpacedRectSide\",\"uuid\":\"38ea75c0-d618-4b9d-8119-0da292fc369a\"}]},\"type\":\"ConnectorPlacement.EquallySpacedConnector\",\"uuid\":\"3f5248e6-8959-4c7a-b37c-028caf22ec16\"}],\"packageUris\":[\"http://schema.mathworks.com/mf0/Connector/R2020b\"],\"version\":\"1.0\"}"
  z_dodot : Subsystem
      settings: PortSchema="{\"entries\":[{\"content\":{\"sides\":[{\"content\":{\"connectorIds\":[\"In1\",\"In2\",\"In3\",\"In4\",\"In5\",\"In6\"]},\"type\":\"ConnectorPlacement.EquallySpacedRectSide\",\"uuid\":\"469c81c2-5293-4bed-8306-2e0ffdc3049a\"},{\"content\":{\"connectorIds\":[\"In7\",\"Out1\"],\"side\":\"RIGHT\"},\"type\":\"ConnectorPlacement.EquallySpacedRectSide\",\"uuid\":\"eb4ccd77-d780-4218-b458-09af15aced4a\"},{\"content\":{\"connectorIds\":[],\"side\":\"TOP\"},\"type\":\"ConnectorPlacement.EquallySpacedRectSide\",\"uuid\":\"6490e6c2-4333-4700-a2fe-e5c918a55a4d\"}]},\"type\":\"ConnectorPlacement.EquallySpacedConnector\",\"uuid\":\"88d53b3a-6da6-4ffe-908b-5dd465569eed\"}],\"packageUris\":[\"http://schema.mathworks.com/mf0/Connector/R2020b\"],\"version\":\"1.0\"}"
  x : Outport
  x_dot : Outport  Port=2
  y : Outport  Port=3
  y_dot : Outport  Port=4
  z : Outport  Port=5
  z_dot : Outport  Port=6
  wires:
  Integrator10/1 -> z_dot/1, z_dodot/7(z_dot), Integrator11/1  "z_dot"
  Integrator8/1 -> Integrator9/1, y_dotdot/8(y_dot), y_dot/1  "y_dot"
  Integrator9/1 -> y/1  "y"
  Integrator7/1 -> x/1  "x"
  Integrator6/1 -> x_dotdot/8(x_dot), x_dot/1, Integrator7/1  "x_dot"
  Integrator11/1 -> z/1  "z"
  U1/1 -> z_dodot/1(U1), y_dotdot/1(U1), x_dotdot/1(U1)  "U1"
  phi/1 -> y_dotdot/2(phi), x_dotdot/2(phi), z_dodot/2(phi)  "Phi"
  theta/1 -> z_dodot/3(theta), y_dotdot/3(theta), x_dotdot/3(theta)  "Theta"
  psi/1 -> y_dotdot/4(psi), x_dotdot/4(psi)  "Psi"
  FWx/1 -> z_dodot/4(FWx), y_dotdot/5(FWx), x_dotdot/5(FWx)  "FWx"
  FWy/1 -> z_dodot/5(FWy), y_dotdot/6(FWy), x_dotdot/6(FWy)  "FWy"
  FWz/1 -> z_dodot/6(FWz), y_dotdot/7(FWz), x_dotdot/7(FWz)  "FWz"
  z_dodot/1(z_dotdot) -> Integrator10/1
  y_dotdot/1(y_dotdot) -> Integrator8/1
  x_dotdot/1(x_dotdot) -> Integrator6/1

== system Quadcopter_State_model_Arduino/Fuzzy Simulation/Quadcopter Dynamics1/Translational Wind Engine ==
  phi : Inport
  theta : Inport  Port=2
  psi : Inport  Port=3
  Projected Areas : Subsystem
  Wind Forces : Subsystem
  Wind Generation : Subsystem
  FWx : Outport
  FWy : Outport  Port=2
  FWz : Outport  Port=3
  wires:
  theta/1 -> Projected Areas/1(theta)
  Wind Generation/3(VWz) -> Wind Forces/6(VWz)
  Projected Areas/3(Az) -> Wind Forces/3(Az)
  Wind Forces/3(FWz) -> FWz/1
  Wind Generation/2(VWy) -> Wind Forces/5(VWy)
  Projected Areas/1(Ax) -> Wind Forces/1(Ax)
  Projected Areas/2(Ay) -> Wind Forces/2(Ay)
  Wind Generation/1(VWx) -> Wind Forces/4(VWx)
  phi/1 -> Projected Areas/3(phi)
  psi/1 -> Projected Areas/2(psi)
  Wind Forces/2(FWy) -> FWy/1
  Wind Forces/1(FWx) -> FWx/1

== system Quadcopter_State_model_Arduino/Fuzzy Simulation/Sensors/Sampling ==
  X_State : Inport
  Memory : Memory
  Square Wave Generator Enable : SignalGenerator  WaveForm=square  Frequency=234  Units=rad/sec
  Switch : Switch  Criteria=u2 > Threshold  SaturateOnIntegerOverflow=off  InputSameDT=off
  X_State Sensor : Outport
  wires:
  Switch/1 -> Memory/1
  Memory/1 -> X_State Sensor/1, Switch/3
  Square Wave Generator Enable/1 -> Switch/2
  X_State/1 -> Switch/1

== system Quadcopter_State_model_Arduino/PID Simulation/Controller_Subsystem/  ==
  phi : Inport
  theta : Inport  Port=2
  psi : Inport  Port=3
  e_x : Inport  Port=4
  e_y : Inport  Port=5
  Attitude Controller : Subsystem
  Saturation : Saturate  UpperLimit=0.3  LowerLimit=-0.3
  Saturation1 : Saturate  UpperLimit=0.3  LowerLimit=-0.3
  Scope : Scope  NumInputPorts=6
  Sum : Sum  Inputs=|+-
  Sum1 : Sum  Inputs=|+-
  World to Body Conversion : Subsystem
  U3 : Outport
  U2 : Outport  Port=2
  wires:
  psi/1 -> World to Body Conversion/3(psi)
  e_y/1 -> World to Body Conversion/1(e_y)
  e_x/1 -> World to Body Conversion/2(e_x)
  World to Body Conversion/1(phi_d) -> Sum/1, Scope/1  "phi_d"
  World to Body Conversion/2(theta_d) -> Scope/2, Sum1/1  "theta_d"
  Attitude Controller/1(U2) -> U2/1
  Attitude Controller/2(U3) -> U3/1
  Sum/1 -> Saturation/1  "e_phi"
  Sum1/1 -> Saturation1/1  "e_theta"
  phi/1 -> Sum/2, Scope/5
  theta/1 -> Scope/6, Sum1/2
  Saturation/1 -> Scope/3, Attitude Controller/1(e_phi)  "e_phi_sat"
  Saturation1/1 -> Scope/4, Attitude Controller/2(e_theta)  "e_theta_sat"

== system Quadcopter_State_model_Arduino/PID Simulation/Controller_Subsystem/Altitude Controller ==
  e_z : Inport
  PID Controller : slpidlib/PID Controller  Controller=PID  Form=Parallel  TimeDomain=Continuous-time  UseExternalTs=off  SampleTime=-1  IntegratorMethod=Forward Euler  FilterMethod=Forward Euler  ControllerParametersSource=internal  P=2  I=1  UseKiTs=off  D=2  N=3.65992  UseFilter=on  TunerSelectOption=Transfer Function Based (PID Tuner App)  InitialConditionSource=internal  InitialConditionForIntegrator=0  InitialConditionForFilter=0  DifferentiatorICPrevScaledInput=0  ExternalReset=none  TrackingMode=off  Kt=1  LimitOutput=off  SatLimitsSource=internal  UpperSaturationLimit=inf  LowerSaturationLimit=-inf  LinearizeAsGain=on  AntiWindupMode=none  Kb=1  POutMin=[]  POutMax=[]  IOutMin=[]  IOutMax=[]  DOutMin=[]  DOutMax=[]  NOutMin=[]  NOutMax=[]  SumOutMin=[]  SumOutMax=[]  SaturationOutMin=[]  SaturationOutMax=[]  PParamMin=[]  PParamMax=[]  IParamMin=[]  IParamMax=[]  DParamMin=[]  DParamMax=[]  NParamMin=[]  NParamMax=[]  KbParamMin=[]  KbParamMax=[]  KtParamMin=[]  KtParamMax=[]  KbOutMin=[]  KbOutMax=[]  KtOutMin=[]  KtOutMax=[]  IntegratorOutMin=[]  IntegratorOutMax=[]  FilterOutMin=[]  FilterOutMax=[]  SumI1OutMin=[]  SumI1OutMax=[]  SumI2OutMin=[]  SumI2OutMax=[]  SumI3OutMin=[]  SumI3OutMax=[]  SumI4OutMin=[]  SumI4OutMax=[]  SumDOutMin=[]  SumDOutMax=[]  DifferentiatorOutMin=[]  DifferentiatorOutMax=[]  FilterDiffOutCoefMin=[]  FilterDiffOutCoefMax=[]  ReciprocalOutMin=[]  ReciprocalOutMax=[]  SumDenOutMin=[]  SumDenOutMax=[]  SumNumOutMin=[]  SumNumOutMax=[]  DivideOutMin=[]  DivideOutMax=[]  UdiffTsProdOutMin=[]  UdiffTsProdOutMax=[]  NTsProdOutMin=[]  NTsProdOutMax=[]  UintegralTsProdOutMin=[]  UintegralTsProdOutMax=[]  UngainTsProdOutMin=[]  UngainTsProdOutMax=[]  ClampingZeroOutDataTypeStr=Inherit: Inherit via back propagation  ClampingZeroOutMin=[]  ClampingZeroOutMax=[]  FilterDenConstantOutDataTypeStr=Inherit: Inherit via back propagation  FilterDenConstantOutMin=[]  FilterDenConstantOutMax=[]  PCopyOutDataTypeStr=Inherit: Inherit via back propagation  PCopyOutMin=[]  PCopyOutMax=[]  NCopyOutDataTypeStr=Inherit: Inherit via back propagation  NCopyOutMin=[]  NCopyOutMax=[]  IntegratorContinuousStateAttributes=''  IntegratorStateMustResolveToSignalObject=off  IntegratorRTWStateStorageClass=Auto  FilterContinuousStateAttributes=''  FilterStateMustResolveToSignalObject=off  FilterRTWStateStorageClass=Auto  ParallelPVariant=InternalParameters  IdealPVariant=Disabled  IVariant=InternalParameters  DVariant=InternalParameters  IntegratorVariant=Continuous  SatVariant=Disabled  AWVariant=Passthrough  PCopyVariant=Disabled  TRVariant=Disabled  FdbkBlocksVariant=Forward  IdealPFdbkVariant=Disabled  SatFdbkVariant=Disabled  DerivativeFilterVariant=ContFilter  NVariant=InternalParameters  NCopyVariant=Disabled  FilterICVariant=InternalICsFilter  IntegratorICVariant=InternalICs  ExternalResetVariant=Disabled  TRSumVariant=Passthrough  SumFdbkVariant=Disabled  SumVariant=Sum_PID  TsampFilterVariant=InternalTs  TsampNgainVariant=Passthrough  TsampIntegralVariant=Passthrough  ExternalSaturationOutDataTypeStr=Inherit: Same as second input  aMode=0
  U1 : Outport
  wires:
  e_z/1 -> PID Controller/1
  PID Controller/1 -> U1/1  "U1"

== system Quadcopter_State_model_Arduino/PID Simulation/Controller_Subsystem/Heading Controller ==
  e_psi : Inport
  Derivative : Derivative
  Gain : Gain  Gain=kd
  Gain1 : Gain  Gain=kp
  Gain2 : Gain  Gain=ki
  Integrator : Integrator
  Sum1 : Sum  Inputs=+++
  U4 : Outport
  wires:
  Derivative/1 -> Sum1/1
  Gain/1 -> Derivative/1
  Sum1/1 -> U4/1  "U4"
  Gain1/1 -> Sum1/2
  e_psi/1 -> Gain2/1, Gain1/1, Gain/1
  Integrator/1 -> Sum1/3
  Gain2/1 -> Integrator/1

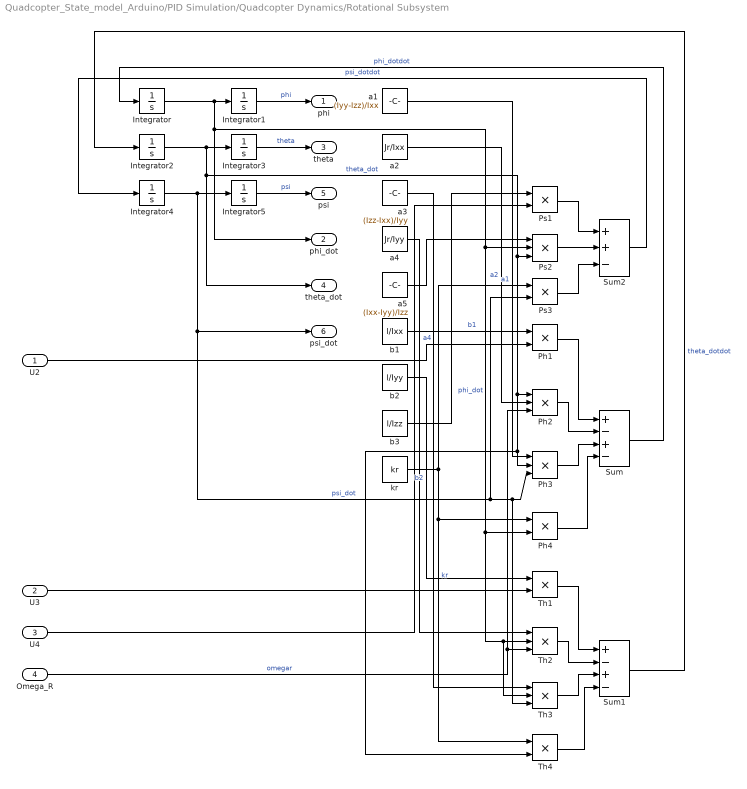
== system Quadcopter_State_model_Arduino/PID Simulation/Quadcopter Dynamics/Rotational Subsystem ==
  U2 : Inport
  U3 : Inport  Port=2
  U4 : Inport  Port=3
  Omega_R : Inport  Port=4
  Integrator{,1..5} (6 alike) : Integrator
  Ph1 : Product
  Ph2 : Product  Inputs=3
  Ph3 : Product  Inputs=3
  Ph4 : Product
  Ps1 : Product
  Ps2 : Product  Inputs=3
  Ps3 : Product
  Sum : Sum  Inputs=+-+-
  Sum1 : Sum  Inputs=+-+-
  Sum2 : Sum  Inputs=++-
  Th1 : Product
  Th2 : Product  Inputs=3
  Th3 : Product  Inputs=3
  Th4 : Product
  a1 : Constant  Value=(Iyy-Izz)/Ixx
  a2 : Constant  Value=Jr/Ixx
  a3 : Constant  Value=(Izz-Ixx)/Iyy
  a4 : Constant  Value=Jr/Iyy
  a5 : Constant  Value=(Ixx-Iyy)/Izz
  b1 : Constant  Value=l/Ixx
  b2 : Constant  Value=l/Iyy
  b3 : Constant  Value=l/Izz
  kr : Constant  Value=kr
  phi : Outport
  phi_dot : Outport  Port=2
  theta : Outport  Port=3
  theta_dot : Outport  Port=4
  psi : Outport  Port=5
  psi_dot : Outport  Port=6
  wires:
  U4/1 -> Ps1/2
  Ph3/1 -> Sum/3
  kr/1 -> Ps3/1, Ph4/1, Th4/1  "kr"
  Th1/1 -> Sum1/1
  Sum/1 -> Integrator/1  "phi_dotdot"
  Omega_R/1 -> Ph2/3, Th2/3  "omegar"
  Th2/1 -> Sum1/2
  Integrator4/1 -> Integrator5/1, psi_dot/1, Ps3/2, Th3/3, Ph3/3  "psi_dot"
  Integrator2/1 -> Integrator3/1, theta_dot/1, Ps2/3, Ph3/2, Th4/2, Ph2/1  "theta_dot"
  Th3/1 -> Sum1/3
  a4/1 -> Th2/1  "a4"
  Sum2/1 -> Integrator4/1  "psi_dotdot"
  Integrator1/1 -> phi/1  "phi"
  U2/1 -> Ph1/2
  Sum1/1 -> Integrator2/1  "theta_dotdot"
  Integrator/1 -> phi_dot/1, Ps2/2, Ph4/2, Th3/2, Th2/2, Integrator1/1  "phi_dot"
  Th4/1 -> Sum1/4
  Integrator3/1 -> theta/1  "theta"
  b1/1 -> Ph1/1  "b1"
  a3/1 -> Th3/1
  b3/1 -> Ps1/1
  a2/1 -> Ph2/2  "a2"
  a1/1 -> Ph3/1  "a1"
  a5/1 -> Ps2/1
  U3/1 -> Th1/2
  Ps3/1 -> Sum2/3
  Ps1/1 -> Sum2/1
  Ps2/1 -> Sum2/2
  Ph4/1 -> Sum/4
  b2/1 -> Th1/1  "b2"
  Ph1/1 -> Sum/1
  Ph2/1 -> Sum/2
  Integrator5/1 -> psi/1  "psi"

== system Quadcopter_State_model_Arduino/PID Simulation/Quadcopter Dynamics/Translational Subsystem 2.0 ==
  U1 : Inport
  phi : Inport  Port=2
  theta : Inport  Port=3
  psi : Inport  Port=4
  FWx : Inport  Port=5
  FWy : Inport  Port=6
  FWz : Inport  Port=7
  Integrator{6..11} (6 alike) : Integrator
  x_dotdot : Subsystem
      settings: PortSchema="{\"entries\":[{\"content\":{\"sides\":[{\"content\":{\"connectorIds\":[\"In1\",\"In2\",\"In3\",\"In4\",\"In5\",\"In6\",\"In7\"]},\"type\":\"ConnectorPlacement.EquallySpacedRectSide\",\"uuid\":\"e18be740-6f58-4938-bfd9-cb9ac7dcd4da\"},{\"content\":{\"connectorIds\":[\"In8\",\"Out1\"],\"side\":\"RIGHT\"},\"type\":\"ConnectorPlacement.EquallySpacedRectSide\",\"uuid\":\"68bb1cbd-6e96-465a-bd08-5b84ec49c8af\"},{\"content\":{\"connectorIds\":[],\"side\":\"TOP\"},\"type\":\"ConnectorPlacement.EquallySpacedRectSide\",\"uuid\":\"38ea75c0-d618-4b9d-8119-0da292fc369a\"}]},\"type\":\"ConnectorPlacement.EquallySpacedConnector\",\"uuid\":\"3f5248e6-8959-4c7a-b37c-028caf22ec16\"}],\"packageUris\":[\"http://schema.mathworks.com/mf0/Connector/R2020b\"],\"version\":\"1.0\"}"
  y_dotdot : Subsystem
      settings: PortSchema="{\"entries\":[{\"content\":{\"sides\":[{\"content\":{\"connectorIds\":[\"In1\",\"In2\",\"In3\",\"In4\",\"In5\",\"In6\",\"In7\"]},\"type\":\"ConnectorPlacement.EquallySpacedRectSide\",\"uuid\":\"e18be740-6f58-4938-bfd9-cb9ac7dcd4da\"},{\"content\":{\"connectorIds\":[\"In8\",\"Out1\"],\"side\":\"RIGHT\"},\"type\":\"ConnectorPlacement.EquallySpacedRectSide\",\"uuid\":\"68bb1cbd-6e96-465a-bd08-5b84ec49c8af\"},{\"content\":{\"connectorIds\":[],\"side\":\"TOP\"},\"type\":\"ConnectorPlacement.EquallySpacedRectSide\",\"uuid\":\"38ea75c0-d618-4b9d-8119-0da292fc369a\"}]},\"type\":\"ConnectorPlacement.EquallySpacedConnector\",\"uuid\":\"3f5248e6-8959-4c7a-b37c-028caf22ec16\"}],\"packageUris\":[\"http://schema.mathworks.com/mf0/Connector/R2020b\"],\"version\":\"1.0\"}"
  z_dodot : Subsystem
      settings: PortSchema="{\"entries\":[{\"content\":{\"sides\":[{\"content\":{\"connectorIds\":[\"In1\",\"In2\",\"In3\",\"In4\",\"In5\",\"In6\"]},\"type\":\"ConnectorPlacement.EquallySpacedRectSide\",\"uuid\":\"469c81c2-5293-4bed-8306-2e0ffdc3049a\"},{\"content\":{\"connectorIds\":[\"In7\",\"Out1\"],\"side\":\"RIGHT\"},\"type\":\"ConnectorPlacement.EquallySpacedRectSide\",\"uuid\":\"eb4ccd77-d780-4218-b458-09af15aced4a\"},{\"content\":{\"connectorIds\":[],\"side\":\"TOP\"},\"type\":\"ConnectorPlacement.EquallySpacedRectSide\",\"uuid\":\"6490e6c2-4333-4700-a2fe-e5c918a55a4d\"}]},\"type\":\"ConnectorPlacement.EquallySpacedConnector\",\"uuid\":\"88d53b3a-6da6-4ffe-908b-5dd465569eed\"}],\"packageUris\":[\"http://schema.mathworks.com/mf0/Connector/R2020b\"],\"version\":\"1.0\"}"
  x : Outport
  x_dot : Outport  Port=2
  y : Outport  Port=3
  y_dot : Outport  Port=4
  z : Outport  Port=5
  z_dot : Outport  Port=6
  wires:
  Integrator10/1 -> z_dot/1, z_dodot/7(z_dot), Integrator11/1  "z_dot"
  Integrator8/1 -> Integrator9/1, y_dotdot/8(y_dot), y_dot/1  "y_dot"
  Integrator9/1 -> y/1  "y"
  Integrator7/1 -> x/1  "x"
  Integrator6/1 -> x_dotdot/8(x_dot), x_dot/1, Integrator7/1  "x_dot"
  Integrator11/1 -> z/1  "z"
  U1/1 -> z_dodot/1(U1), y_dotdot/1(U1), x_dotdot/1(U1)  "U1"
  phi/1 -> y_dotdot/2(phi), x_dotdot/2(phi), z_dodot/2(phi)  "Phi"
  theta/1 -> z_dodot/3(theta), y_dotdot/3(theta), x_dotdot/3(theta)  "Theta"
  psi/1 -> y_dotdot/4(psi), x_dotdot/4(psi)  "Psi"
  FWx/1 -> z_dodot/4(FWx), y_dotdot/5(FWx), x_dotdot/5(FWx)  "FWx"
  FWy/1 -> z_dodot/5(FWy), y_dotdot/6(FWy), x_dotdot/6(FWy)  "FWy"
  FWz/1 -> z_dodot/6(FWz), y_dotdot/7(FWz), x_dotdot/7(FWz)  "FWz"
  z_dodot/1(z_dotdot) -> Integrator10/1
  y_dotdot/1(y_dotdot) -> Integrator8/1
  x_dotdot/1(x_dotdot) -> Integrator6/1

== system Quadcopter_State_model_Arduino/PID Simulation/Quadcopter Dynamics/Translational Wind Engine ==
  phi : Inport
  theta : Inport  Port=2
  psi : Inport  Port=3
  Projected Areas : Subsystem
  Wind Forces : Subsystem
  Wind Generation : Subsystem
  FWx : Outport
  FWy : Outport  Port=2
  FWz : Outport  Port=3
  wires:
  theta/1 -> Projected Areas/1(theta)
  Wind Generation/3(VWz) -> Wind Forces/6(VWz)
  Projected Areas/3(Az) -> Wind Forces/3(Az)
  Wind Forces/3(FWz) -> FWz/1
  Wind Generation/2(VWy) -> Wind Forces/5(VWy)
  Projected Areas/1(Ax) -> Wind Forces/1(Ax)
  Projected Areas/2(Ay) -> Wind Forces/2(Ay)
  Wind Generation/1(VWx) -> Wind Forces/4(VWx)
  phi/1 -> Projected Areas/3(phi)
  psi/1 -> Projected Areas/2(psi)
  Wind Forces/2(FWy) -> FWy/1
  Wind Forces/1(FWx) -> FWx/1

== system Quadcopter_State_model_Arduino/PID Simulation/Sensors/Noise Generator ==
  note: Bus is split to allow generation of different
      | noise on different readings if desired
  X_State : Inport
  Bus Creator : BusCreator  Inputs=12
  Bus Selector : BusSelector  OutputSignals=phi,phi_dot,theta,theta_dot,psi,psi_dot,x,x_dot,y,y_dot,z,z_dot
  Noise : RandomNumber  Variance=.01  SampleTime=1
  Sum{,1..11} (12 alike) : Sum
  Waveform Generator1 : simulink/Sources/Waveform Generator  OutMin=[]  OutMax=[]  OutDataTypeStr=double  SelectedSignal=1  Signals=sin(0.01,3,1)  BlockNames=MultiportSwitch_3635ecf662dd4f1  SampleTime=0.1
  X_State_Noisy : Outport
  wires:
  Bus Selector/11 -> Sum10/1  "<z>"
  Bus Selector/10 -> Sum9/1  "<y_dot>"
  Bus Selector/5 -> Sum4/1  "<psi>"
  Bus Selector/4 -> Sum3/1  "<theta_dot>"
  Sum4/1 -> Bus Creator/5  "psi"
  Noise/1 -> Sum10/2, Sum11/2, Sum9/2, Sum8/2, Sum7/2, Sum6/2, Sum5/2, Sum4/2, Sum3/2, Sum2/2, Sum1/2, Sum/2
  Bus Selector/8 -> Sum7/1  "<x_dot>"
  Bus Selector/7 -> Sum6/1  "<x>"
  Bus Selector/9 -> Sum8/1  "<y>"
  Sum10/1 -> Bus Creator/11  "z"
  Bus Selector/3 -> Sum2/1  "<theta>"
  Bus Selector/12 -> Sum11/1  "<z_dot>"
  Bus Selector/2 -> Sum1/1  "<phi_dot>"
  Sum/1 -> Bus Creator/1  "phi"
  Bus Selector/1 -> Sum/1  "<phi>"
  Sum2/1 -> Bus Creator/3  "theta"
  Bus Selector/6 -> Sum5/1  "<psi_dot>"
  Sum9/1 -> Bus Creator/10  "y_dot"
  Sum5/1 -> Bus Creator/6  "psi_dot"
  Sum7/1 -> Bus Creator/8  "x_dot"
  Sum1/1 -> Bus Creator/2  "phi_dot"
  Sum3/1 -> Bus Creator/4  "theta_dot"
  Sum8/1 -> Bus Creator/9  "y"
  Sum11/1 -> Bus Creator/12  "z_dot"
  Sum6/1 -> Bus Creator/7  "x"
  X_State/1 -> Bus Selector/1
  Bus Creator/1 -> X_State_Noisy/1  "X_State_Noisy"
